simulink model "Simulation_half_bridge_with_LC_filter"  (R2020b)
settings: Solver=ode23tb  StartTime=0.0  StopTime=stop_time  MaxStep=max_step_size  RelTol=tolerance  EnableMultiTasking=on
values from neighbouring files (symbols this model uses):
  D_ref = D * 100    (= 75)    [init_cstes.m]    (also in init_cstes_filter.m)
  Dead_time = 10e-6    (= 1e-05)    [init_cstes.m]    (also in init_cstes_filter.m)
  f_sw = 2e3    (= 2000)    [init_cstes.m]    (also in init_cstes_IGBT.m; init_cstes_filter.m)
  filter_C = facteur * 1e-3    (= 0.01)    [init_cstes_filter.m]
  filter_L = facteur * 0.3e-3    (= 0.003)    [init_cstes_filter.m]
  PWM_period = 1/f_sw    (= 0.0005)    [init_cstes.m]    (also in init_cstes_filter.m)
  R_i = 1e-6    (= 1e-06)    [init_cstes.m]    (also in init_cstes_IGBT.m; init_cstes_filter.m)
  RLE_E = 140    [init_cstes.m]    (also in init_cstes_filter.m)
  RLE_L = 10e-3    (= 0.01)    [init_cstes.m]    (also in init_cstes_filter.m)
  RLE_R = 0.2    [init_cstes.m]    (also in init_cstes_filter.m)
  V_AN_ref = V_ref    (= 150)    [init_cstes.m]    (also in init_cstes_filter.m)
  V_b = 200    [init_cstes.m]    (also in init_cstes_IGBT.m; init_cstes_filter.m)
libraries: powerlib x15, powerlib_meascontrol x4, simulink x1
settings Model: Creator=ULB  LastModifiedBy=arnaudsaison
settings SolverCC: SolverResetMethod=Robust
settings DataIOCC: LimitDataPoints=on  SaveFormat=Array  SignalLoggingSaveFormat=ModelDataLogs  ReturnWorkspaceOutputs=off
settings OptimizationCC: ExpressionDepthLimit=2147483647  LifeSpan=inf
settings DebuggingCC: UnderspecifiedInitializationDetection=Classic  MergeDetectMultiDrivingBlocksExec=none  SolverPrmCheckMsg=warning  FcnCallInpInsideContextMsg=warning  UnconnectedInputMsg=none  UnconnectedOutputMsg=none  UnconnectedLineMsg=none  StateNameClashWarn=warning  SFUnexpectedBacktrackingDiag=warning  SFNoUnconditionalDefaultTransitionDiag=warning  SFExecutionAtInitializationDiag=none  ArithmeticOperatorsInVariantConditions=warning
settings HardwareCC: ProdBitPerPointer=32  ProdBitPerSizeT=32  ProdBitPerPtrDiffT=32  ProdLargestAtomicFloat=None  ProdIntDivRoundTo=Undefined  ProdEndianess=Unspecified  ProdWordSize=32  ProdHWDeviceType=32-bit Generic
settings ModelReferenceCC: PropagateSignalLabelsOutOfModel=off
settings SFSimCC: SimUseLocalCustomCode=off  CustomCodeUndefinedFunction=UseInterfaceOnly
settings RTWCC: RTWUseLocalCustomCode=off
settings CodeAppCC: StateflowObjectComments=on
settings GRTTargetCC: TargetLangStandard=C89/C90 (ANSI)  CombineOutputUpdateFcns=off  GRTInterface=on
settings ConfigComp: CovMetricSettings=dw  CovSaveCumulativeToWorkspaceVar=on  CovSaveSingleToWorkspaceVar=on  CovExternalEMLEnable=off
settings SimscapeCC: SimscapeNormalizeSystem=off

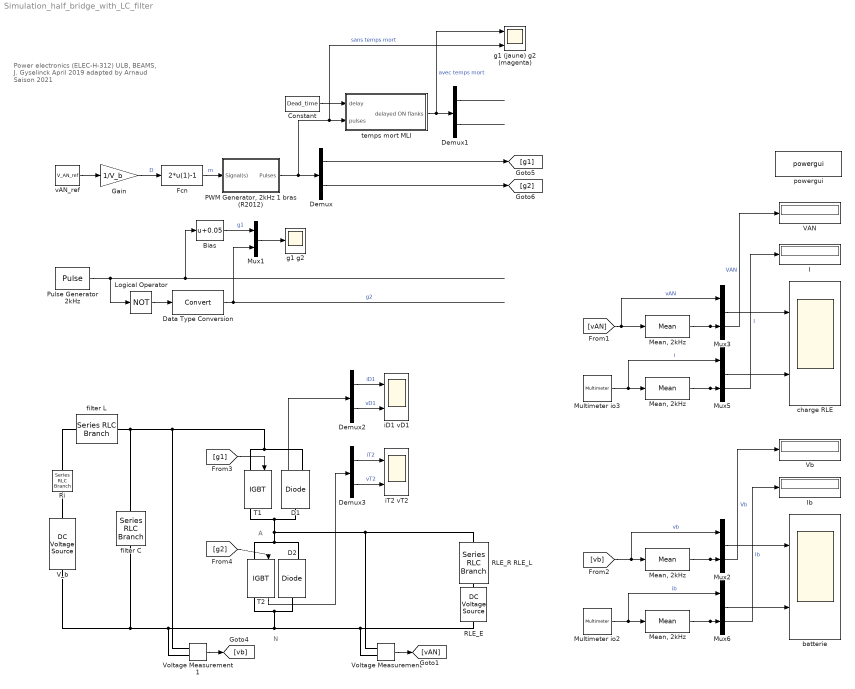
== system Simulation_half_bridge_with_LC_filter ==
  note: A
  note: N
  note: Power electronics (ELEC-H-312)
      | ULB, BEAMS, J. Gyselinck April 2019
      | adapted by Arnaud Saison 2021
  "   Mean, 2kHz   " : powerlib_meascontrol/Measurements/Mean  Freq=f_sw  Vinit=0  Ts=0
  "  Mean, 2kHz " : powerlib_meascontrol/Measurements/Mean  Freq=f_sw  Vinit=0  Ts=0
  "  Mean, 2kHz  " : powerlib_meascontrol/Measurements/Mean  Freq=f_sw  Vinit=0  Ts=0
  Bias : Bias  Bias=0.05
  Constant : Constant  Value=Dead_time
  D1 : powerlib/Power Electronics/Diode  Ron=0.001  Lon=0  Vf=0.8  IC=0  UseSnubber=off  Rs=500  Cs=250e-9  Measurements=on
  D2 : powerlib/Power Electronics/Diode  Ron=0.001  Lon=0  Vf=0.8  IC=0  UseSnubber=off  Rs=500  Cs=250e-9  Measurements=on
  Data Type Conversion : DataTypeConversion
  Demux{,1..3} (4 alike) : Demux  Outputs=2
  Fcn : Fcn  Expr=2*u(1)-1
  Gain : Gain  Gain=1/V_b
  I : Display
      settings: Format=short_e
  Ib : Display
      settings: Format=short_e
  Logical Operator : Logic  Operator=NOT  AllPortsSameDT=off  OutDataTypeStr=boolean
  "Mean, 2kHz" : powerlib_meascontrol/Measurements/Mean  Freq=f_sw  Vinit=0  Ts=0
  Multimeter io2 : powerlib/Measurements/Multimeter  PhasorSimulation=off  OutputType=Complex  sel=6  L=8  Gain=1  yselected={'Ib: Ri'};  PSBOutputType=1  PSBequivalent=0  AxesSetting=[0,0.1,-100,100]  Display=0  SavedBlockNames=-11
  Multimeter io3 : powerlib/Measurements/Multimeter  PhasorSimulation=off  OutputType=Complex  sel=5  L=8  Gain=1  yselected={'Ib: RLE_R RLE_L'};  PSBOutputType=1  PSBequivalent=0  AxesSetting=[0,0.1,-100,100]  Display=0  SavedBlockNames=-11
  Mux{1..3,5..6} (5 alike) : Mux  Inputs=2
  "PWM Generator, 2kHz 1 bras (R2012)" : Subsystem  AncestorBlock="powerlib_extras/Control  Blocks/PWM Generator"  DialogController=POWERSYS.PowerSysDialog  mask(PWM Generator){GeneratorMode=1-arm  bridge (2 pulses), Fc=f_sw, Internal=off, mIndex=0.4, Freq=60, Phase=0}
      mask prompts: GeneratorMode "Generator Mode"; Fc "Carrier frequency (Hz):"; Internal "Internal generation of modulating signal(s)"; mIndex "Modulation index  (0<m<1) :"; Freq "Frequency of output voltage (Hz)"; Phase "Phase of output voltage (degrees)"
      mask help:
      | This block generates pulses for carrier-based PWM (Pulse Width Modulation), self-commutated IGBTs,GTOs or FETs bridges.
      |
      | Depending on the number of bridge arms selected in the "Generator Mode" parameter, the block can be used either for single-phase or three-phase PWM control.
      mask init:
      | if Freq==0
      |     Phase=90;
      | end
      | switch GeneratorMode
      | case 1,
      |     Internal_Phase=0;
      |    Signal_PortWidth=1;
      |    Select1_Elements=[1 2];
      |    Select1_PortWidth=2;
      |    Select3_Elements=[1 2];
      |    Select3_PortWidth=4;
      | case 2,
      |     Internal_Phase=0;
      |     Signal_PortWidth=1;
      |     Select1_Elements=[1 2];
      |     Select1_PortWidth=2;
      |     Select3_Elements=[1 2 3 4];
      |     Select3_PortWidth=4;
      | case 3,
      |     Internal_Phase=[0 -2*pi/3 2*pi/3];
      |     Signal_PortWidth=3;
      |     Select1_Elements=[1 4 2 5 3 6];
      |     Select1_PortWidth=6;
      |    Select3_Elements=[1 2 3 4 5 6];
      |    Select3_PortWidth=12;
      | case 4,
      |     Internal_Phase=[0 -2*pi/3 2*pi/3];
      |     Signal_PortWidth=3;
      |     Select1_Elements=[1 4 2 5 3 6];
      |     Select1_PortWidth=6;
      |    Select3_Elements=[1 2 3 4 5 6 7 8 9 10 11 12];
      |    Select3_PortWidth=12;
      | end
      | power_initmask();
      mask Help: web(psbhelp)
      mask TypeOptions GeneratorMode: 1-arm  bridge (2 pulses) | 2-arm  bridge (4 pulses) | 3-arm  bridge (6 pulses) | Double 3-arm  bridges (12 pulses)
      mask Callback Internal: p3=get_param(gcb,'Internal');if strcmp(p3,'on');visible={'on','on','on','on','on','on'};else;visible={'on','on','on','off','off','off'};end;set_param(gcb,'MaskVisibilities',visible)
  Pulse Generator 2kHz : DiscretePulseGenerator  PulseType=Time based  Period=PWM_period  PulseWidth=D_ref
  RLE_E : powerlib/Electrical Sources/DC Voltage Source  Amplitude=RLE_E  Measurements=None
  RLE_R RLE_L : powerlib/Elements/Series RLC Branch  LConnTagsString=__new0  RConnTagsString=__new0  BranchType=RL  Resistance=RLE_R  Inductance=RLE_L  SetiL0=off  InitialCurrent=0  Capacitance=1e-6  Setx0=off  InitialVoltage=0  Measurements=Branch voltage and current
  Ri : powerlib/Elements/Series RLC Branch  LConnTagsString=__new0  RConnTagsString=__new0  BranchType=R  Resistance=R_i  Inductance=2e-3  SetiL0=off  InitialCurrent=0  Capacitance=1e-6  Setx0=off  InitialVoltage=0  Measurements=Branch voltage and current
  T1 : powerlib/Power Electronics/IGBT  Ron=0.001  Lon=0  Vf=1  Tf=1e-6  Tt=2e-6  IC=0  Rs=1e5  Cs=inf  Measurements=on
  T2 : powerlib/Power Electronics/IGBT  Ron=0.001  Lon=0  Vf=1  Tf=1e-6  Tt=2e-6  IC=0  Rs=1e5  Cs=inf  Measurements=on
  VAN : Display
      settings: Format=short_e
  V_b : powerlib/Electrical Sources/DC Voltage Source  Amplitude=V_b  Measurements=None
  Vb : Display
      settings: Format=short_e
  Voltage Measurement : powerlib/Measurements/Voltage Measurement  PhasorSimulation=off  OutputType=Complex  PSBequivalent=0
  Voltage Measurement1 : powerlib/Measurements/Voltage Measurement  PhasorSimulation=off  OutputType=Complex  PSBequivalent=0
  batterie : Scope  NumInputPorts=2
  charge RLE : Scope  NumInputPorts=2
  filter C : powerlib/Elements/Series RLC Branch  LConnTagsString=__new0  RConnTagsString=__new0  BranchType=C  Resistance=1  Inductance=2e-3  SetiL0=off  InitialCurrent=0  Capacitance=filter_C  Setx0=off  InitialVoltage=200  Measurements=Branch voltage and current
  filter L : powerlib/Elements/Series RLC Branch  LConnTagsString=__new0  RConnTagsString=__new0  BranchType=L  Resistance=0.2  Inductance=filter_L  SetiL0=off  InitialCurrent=0  Capacitance=1e-6  Setx0=off  InitialVoltage=0  Measurements=Branch voltage and current
  g1 (jaune) g2 (magenta) : Scope  NumInputPorts=2
  g1 g2 : Scope
  iD1 vD1 : Scope  NumInputPorts=2
  iT2 vT2 : Scope  NumInputPorts=2
  powergui : powerlib/powergui  SimulationMode=Continuous  SampleTime=1e-6  frequency=60  Iterations=50  frequencyindice=0  Pbase=100e6  ErrMax=1e-4  UnitsV=kV  UnitsW=MW  buscounter=0  FunctionMessages=off  echomessages=off  EnableUseOfTLC=off  CurrentSourceSwitches=off  DisableSnubberDevices=off  DisableRonSwitches=on  DisableVfSwitches=on  DisplayEquations=off  AutomaticDiscreteSolvers=off  SolverType=Tustin  Interpol=off  ExternalGateDelay=off  methode=off  Ts=0  x0status=blocks  SPID=off  SwTol=0  HookPort=off  NonlinearTolerance=1e-4  nMaxIteration=100  ContinueOnMaxIteration=off  RestoreLinks=warning  ResistiveCurrentMeasurement=off  Frange=[0:2:500]  Ylog=off  Xlog=on  ShowGrid=off  save=off  variable=ZData  structure=vio  ZoomFFT=off  StartTime=0.1  cycles=3  DisplayStyle=4  fundamental=50  FreqAxis=off  MaxFrequency=3000  frequencyindicesteady=1  RmsSteady=1  display=off
  temps mort MLI : Subsystem
  vAN_ref : Constant  Value=V_AN_ref
  wires:
  Pulse Generator 2kHz/1 -> Logical Operator/1, Bias/1
  Voltage Measurement/1 -> [vAN]
  Voltage Measurement1/1 -> [vb]
  [g1] -> T1/1
  [g2] -> T2/1
  Logical Operator/1 -> Data Type Conversion/1
  Bias/1 -> Mux1/1  "g1"
  Mux1/1 -> g1 g2/1
  Data Type Conversion/1 -> Mux1/2  "g2"
  Gain/1 -> Fcn/1  "D"
  vAN_ref/1 -> Gain/1
  Constant/1 -> temps mort MLI/1(delay)
  "PWM Generator, 2kHz 1 bras (R2012)"/1(Pulses) -> Demux/1, temps mort MLI/2(pulses), g1 (jaune) g2 (magenta)/2  "sans temps mort"
  temps mort MLI/1(delayed ON flanks) -> Demux1/1, g1 (jaune) g2 (magenta)/1  "avec temps mort"
  Fcn/1 -> "PWM Generator, 2kHz 1 bras (R2012)"/1(Signal(s))  "m"
  Demux2/2 -> iD1 vD1/2  "vD1"
  Demux1/1 -> ?
  Demux1/2 -> ?
  Demux2/1 -> iD1 vD1/1  "iD1"
  Demux/1 -> [g1]
  Demux/2 -> [g2]
  Demux3/2 -> iT2 vT2/2  "vT2"
  Demux3/1 -> iT2 vT2/1  "iT2"
  [vAN] -> Mux3/1, "  Mean, 2kHz "/1  "vAN"
  Mux3/1 -> charge RLE/1
  Multimeter io3/1 -> "Mean, 2kHz"/1, Mux5/1  "i"
  "  Mean, 2kHz "/1 -> VAN/1, Mux3/2  "VAN"
  Mux5/1 -> charge RLE/2
  "Mean, 2kHz"/1 -> I/1, Mux5/2  "I"
  [vb] -> Mux2/1, "  Mean, 2kHz  "/1  "vb"
  Mux2/1 -> batterie/1
  Multimeter io2/1 -> "   Mean, 2kHz   "/1, Mux6/1  "ib"
  "  Mean, 2kHz  "/1 -> Vb/1, Mux2/2  "Vb"
  Mux6/1 -> batterie/2
  "   Mean, 2kHz   "/1 -> Mux6/2, Ib/1  "Ib"
  D1/1 -> Demux2/1
  T2/1 -> Demux3/1
  connections:
  D2/RConn1 -- T2/LConn1 -- Voltage Measurement/LConn1 -- RLE_R RLE_L/LConn1 -- T1/RConn1 -- D1/LConn1
  filter C/RConn1 -- D2/LConn1 -- T2/RConn1 -- Voltage Measurement/LConn2 -- RLE_E/LConn1 -- Voltage Measurement1/LConn2 -- V_b/LConn1
  RLE_E/RConn1 -- RLE_R RLE_L/RConn1
  Voltage Measurement1/LConn1 -- filter L/LConn1 -- filter C/LConn1 -- D1/RConn1 -- T1/LConn1
  Ri/LConn1 -- V_b/RConn1
  Ri/RConn1 -- filter L/RConn1

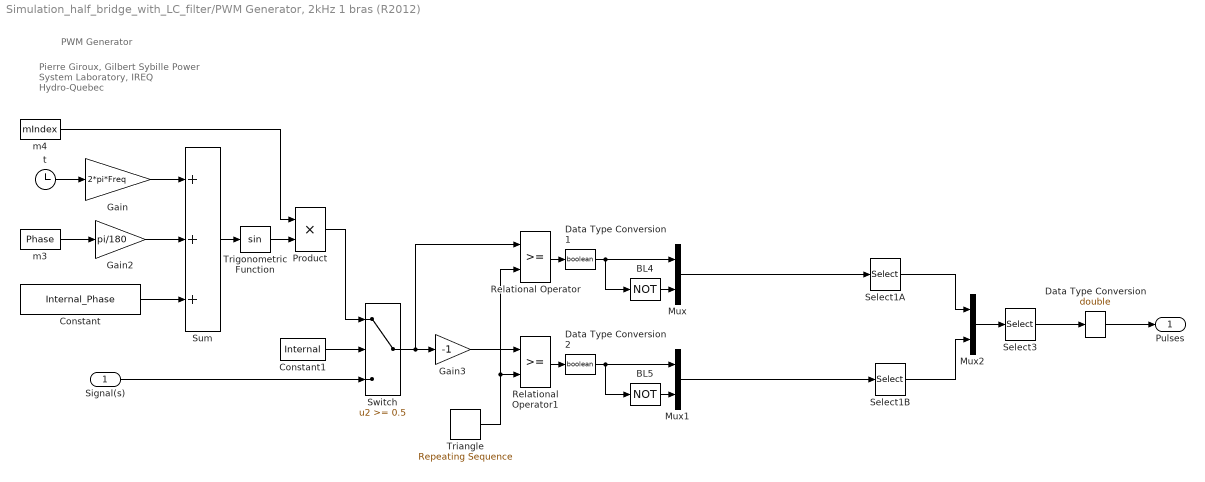
== system Simulation_half_bridge_with_LC_filter/PWM Generator, 2kHz 1 bras (R2012) ==
  note: PWM Generator
  note: Pierre Giroux, Gilbert Sybille
      | Power System Laboratory, IREQ
      | Hydro-Quebec
  Signal(s) : Inport  PortDimensions=Signal_PortWidth
  BL4 : Logic  Operator=NOT  Inputs=1
  BL5 : Logic  Operator=NOT  Inputs=1
  Constant : Constant  Value=Internal_Phase
  Constant1 : Constant  Value=Internal
  Data Type Conversion : DataTypeConversion  OutDataTypeStr=double  SaturateOnIntegerOverflow=on  RndMeth=Zero
  Data Type Conversion1 : DataTypeConversion  OutDataTypeStr=boolean  SaturateOnIntegerOverflow=on  RndMeth=Zero
  Data Type Conversion2 : DataTypeConversion  OutDataTypeStr=boolean  SaturateOnIntegerOverflow=on  RndMeth=Zero
  Gain : Gain  Gain=2*pi*Freq  SaturateOnIntegerOverflow=on  OutDataTypeStr=Inherit: Same as input  ParamDataTypeStr=Inherit: Same as input
  Gain2 : Gain  Gain=pi/180  SaturateOnIntegerOverflow=on  OutDataTypeStr=Inherit: Same as input  ParamDataTypeStr=Inherit: Same as input
  Gain3 : Gain  Gain=-1  SaturateOnIntegerOverflow=on  OutDataTypeStr=Inherit: Same as input  ParamDataTypeStr=Inherit: Same as input
  Mux : Mux  Inputs=2
  Mux1 : Mux  Inputs=2
  Mux2 : Mux  Inputs=2
  Product : Product  InputSameDT=on  SaturateOnIntegerOverflow=on  OutDataTypeStr=Inherit: Same as first input
  Relational Operator : RelationalOperator  RndMeth=Nearest  InputSameDT=on
  Relational Operator1 : RelationalOperator  RndMeth=Nearest  InputSameDT=on
  Select1A : Selector  InputPortWidth=Select1_PortWidth  IndexOptions=Index vector (dialog)  Indices=Select1_Elements  OutputSizes=1
  Select1B : Selector  InputPortWidth=Select1_PortWidth  IndexOptions=Index vector (dialog)  Indices=Select1_Elements  OutputSizes=1
  Select3 : Selector  InputPortWidth=Select3_PortWidth  IndexOptions=Index vector (dialog)  Indices=Select3_Elements  OutputSizes=1
  Sum : Sum  Inputs=+++  InputSameDT=on  SaturateOnIntegerOverflow=on  OutDataTypeStr=Inherit: Same as first input
  Switch : Switch  Threshold=0.5  InputSameDT=on
  Triangle : simulink/Sources/Repeating Sequence  rep_seq_t=[0 1/Fc/4 3/Fc/4 1/Fc]  rep_seq_y=[0 -1 1 0]
  Trigonometric Function : Trigonometry
  m3 : Constant  Value=Phase
  m4 : Constant  Value=mIndex
  t : Clock
  Pulses : Outport  VectorParamsAs1DForOutWhenUnconnected=off
  wires:
  Data Type Conversion2/1 -> Mux1/1, BL5/1
  Relational Operator1/1 -> Data Type Conversion2/1
  Data Type Conversion1/1 -> Mux/1, BL4/1
  Relational Operator/1 -> Data Type Conversion1/1
  Data Type Conversion/1 -> Pulses/1
  Select3/1 -> Data Type Conversion/1
  t/1 -> Gain/1
  Gain/1 -> Sum/1
  Gain2/1 -> Sum/2
  m3/1 -> Gain2/1
  Constant/1 -> Sum/3
  m4/1 -> Product/1
  Sum/1 -> Trigonometric Function/1
  Trigonometric Function/1 -> Product/2
  Signal(s)/1 -> Switch/3
  Constant1/1 -> Switch/2
  Product/1 -> Switch/1
  Gain3/1 -> Relational Operator1/1
  BL4/1 -> Mux/2
  BL5/1 -> Mux1/2
  Mux/1 -> Select1A/1
  Mux1/1 -> Select1B/1
  Select1A/1 -> Mux2/1
  Select1B/1 -> Mux2/2
  Mux2/1 -> Select3/1
  Switch/1 -> Gain3/1, Relational Operator/1
  Triangle/1 -> Relational Operator1/2, Relational Operator/2

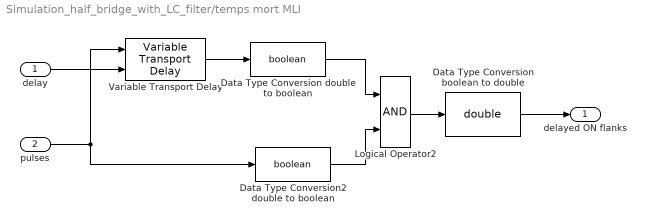
== system Simulation_half_bridge_with_LC_filter/temps mort MLI ==
  delay : Inport
  pulses : Inport  Port=2
  Data Type Conversion boolean to double : DataTypeConversion  OutDataTypeStr=double  SaturateOnIntegerOverflow=on  RndMeth=Zero
  Data Type Conversion double to boolean : DataTypeConversion  OutDataTypeStr=boolean
  Data Type Conversion2 double to boolean : DataTypeConversion  OutDataTypeStr=boolean
  Logical Operator2 : Logic  AllPortsSameDT=off  OutDataTypeStr=boolean
  Variable Transport Delay : VariableTransportDelay  VariableDelayType=Variable transport delay  MaximumDelay=10
  delayed ON flanks : Outport  VectorParamsAs1DForOutWhenUnconnected=off
  wires:
  Data Type Conversion boolean to double/1 -> delayed ON flanks/1
  delay/1 -> Variable Transport Delay/2
  Logical Operator2/1 -> Data Type Conversion boolean to double/1
  pulses/1 -> Data Type Conversion2 double to boolean/1, Variable Transport Delay/1
  Data Type Conversion2 double to boolean/1 -> Logical Operator2/2
  Data Type Conversion double to boolean/1 -> Logical Operator2/1
  Variable Transport Delay/1 -> Data Type Conversion double to boolean/1
